simulink model "Motor_dc"  (R2016a)
settings: Solver=ode15s  StartTime=0.0  StopTime=10  RelTol=1e-3
values from neighbouring files (symbols this model uses):
  b = 0.21372    [Parameter_estimated_Motor.m]    (also in test.m)
  I = 0.0012454    [Parameter_estimated_Motor.m]    (also in test.m)
  Ke = 0.23773    [Parameter_estimated_Motor.m]    (also in test.m)
  Kt = 0.72069    [Parameter_estimated_Motor.m]    (also in test.m)
  L = 0.24427    [Parameter_estimated_Motor.m]    (also in test.m)
  R = 0.97384    [Parameter_estimated_Motor.m]    (also in test.m)
settings Model: Creator=xp  LastModifiedBy=Maha
settings DataIOCC: LimitDataPoints=on  SaveFormat=Array
settings DebuggingCC: SolverPrmCheckMsg=warning
settings HardwareCC: ProdBitPerPointer=32  ProdLargestAtomicFloat=None  ProdIntDivRoundTo=Undefined  ProdEndianess=Unspecified  ProdWordSize=32  ProdHWDeviceType=32-bit Generic
settings ModelReferenceCC: PropagateSignalLabelsOutOfModel=off
settings ConfigComp: CovModelRefEnable=Off  CovSFcnEnable=off

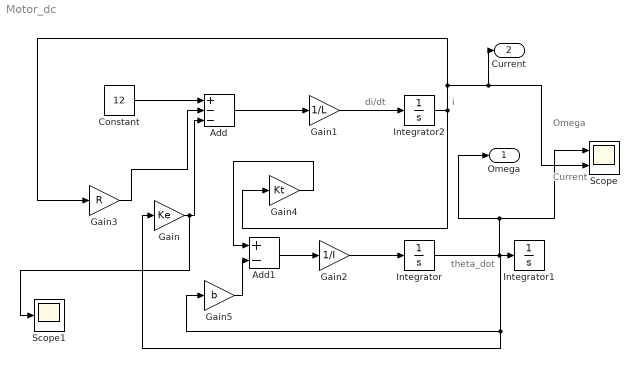
== system Motor_dc ==
  note: Current
  note: Omega
  note: i
  note: di/dt
  note: theta_dot
  Add : Sum  Inputs=+--
  Add1 : Sum  Inputs=+-
  Constant : Constant  Value=12
  Gain : Gain  Gain=Ke
  Gain1 : Gain  Gain=1/L
  Gain2 : Gain  Gain=1/I
  Gain3 : Gain  Gain=R
  Gain4 : Gain  Gain=Kt
  Gain5 : Gain  Gain=b
  Integrator : Integrator
  Integrator1 : Integrator
  Integrator2 : Integrator
  Scope : Scope  NumInputPorts=2
  Scope1 : Scope
  Omega : Outport
  "Current " : Outport  Port=2
  wires:
  Integrator/1 -> Omega/1, Scope/1, Gain/1, Gain5/1, Integrator1/1
  Add/1 -> Gain1/1
  Gain1/1 -> Integrator2/1
  Gain2/1 -> Integrator/1
  Gain/1 -> Scope1/1, Add/3
  Gain3/1 -> Add/2
  Add1/1 -> Gain2/1
  Integrator2/1 -> "Current "/1, Scope/2, Gain3/1, Gain4/1
  Gain4/1 -> Add1/1
  Gain5/1 -> Add1/2
  Constant/1 -> Add/1
